simulink model "State_space_validation_lqr_3_5_2_a"  (R2024b)
settings: Solver=FixedStepAuto  StartTime=0.0  StopTime=20  FixedStep=0.001  RelTol=1e-3
undefined symbols (not defined in the file): degs2rpm, DiscIntNeverNeededParam, K, Kff, National_Instruments, PCI, rdp, rpm2rads, sens, step_gain, Ts, u_bar_max
libraries: sldrtlib x3, simulink x1
settings Model: SimulationMode=external  ExtModeTrigDuration=50001  ExtModeTrigDurationFloating=50001  Creator=perondavid  LastModifiedBy=Enrico
settings DataIOCC: LoggingToFile=on
settings OptimizationCC: ReuseModelBlockBuffer=off
settings HardwareCC: ProdBitPerLong=64  ProdHWDeviceType=Intel->x86-64 (Linux 64)
settings RTWCC: Description=Simulink Desktop Real-Time  SystemTargetFile=sldrt.tlc  TemplateMakefile=sldrt.tmf  RTWCompilerOptimization=on  GPUComputeCapability=3.5
settings CodeAppCC: MaxIdLength=95
settings SimulinkDesktopRealTimeCC: TargetLibSuffix=_sldrt.a  TargetPreCompLibLocation=D:\Programmi (D)\MATLAB\R2024b\toolbox\sldrt\lib\win64  ParMdlRefBuildCompliant=on

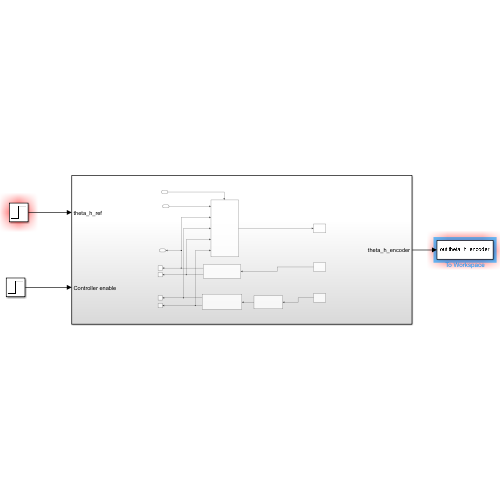
[thumbnail: Simulink's stored preview of the top-level diagram]
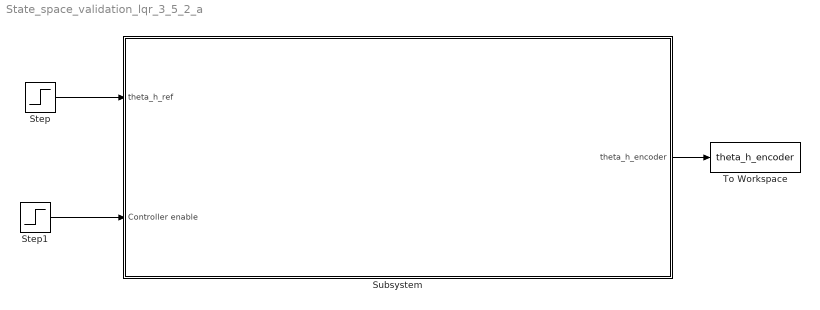
== system State_space_validation_lqr_3_5_2_a ==
  Step : Step  Time=3  After=step_gain  SampleTime=0
  Step1 : Step  Time=2  SampleTime=0
  Subsystem : Subsystem
  To Workspace : ToWorkspace  VariableName=theta_h_encoder  SaveFormat=Structure With Time  SampleTime=Ts
  wires:
  Step/1 -> Subsystem/1(theta_h_ref)
  Step1/1 -> Subsystem/2(Controller enable)
  Subsystem/1(theta_h_encoder) -> To Workspace/1

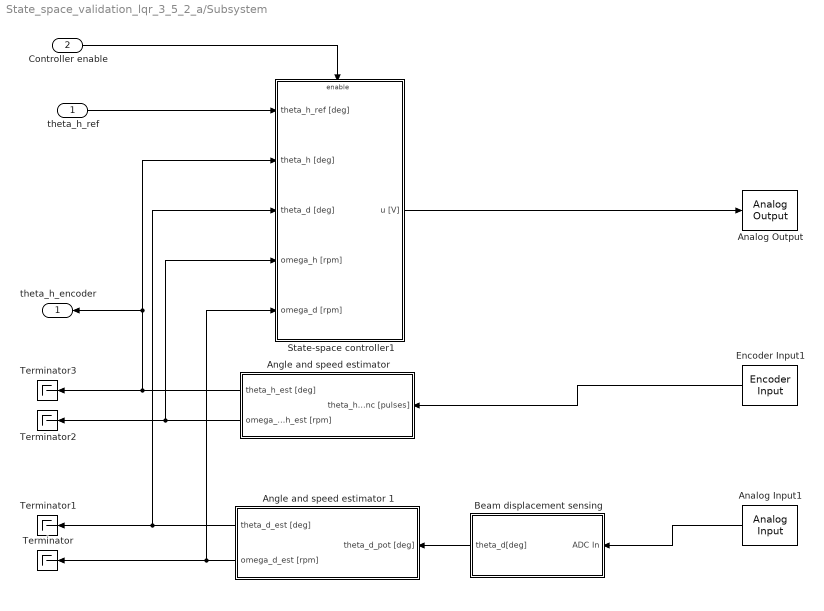
== system State_space_validation_lqr_3_5_2_a/Subsystem ==
  theta_h_ref : Inport
  Controller enable : Inport  Port=2
  Analog Input1 : sldrtlib/Analog Input  SampleTime=-1  MaxMissedTicks=10  ShowMissedTicks=off  YieldWhenWaiting=off  DrvName=National_Instruments/PCI-6221  DrvAddress=4294967295  DrvOptions=[0 0 0 2 0]  Channels=[3, 4]  RangeMode=1  VoltRange=2  DataType=1
      settings: AttributesFormatString=National Instruments\nPCI-6221 [auto]
  Analog Output : sldrtlib/Analog Output  SampleTime=-1  MaxMissedTicks=10  ShowMissedTicks=off  YieldWhenWaiting=off  DrvName=National_Instruments/PCI-6221  DrvAddress=4294967295  DrvOptions=[0 0 0 2 0]  Channels=1  RangeMode=1  VoltRange=1  InitialValue=0  FinalValue=0
      settings: AttributesFormatString=National Instruments\nPCI-6221 [auto]
  Angle and speed estimator : Subsystem
  Angle and speed estimator 1 : Subsystem
  Beam displacement sensing : Subsystem
  Encoder Input1 : sldrtlib/Encoder Input  SampleTime=-1  MaxMissedTicks=10  ShowMissedTicks=off  YieldWhenWaiting=off  DrvName=National_Instruments/PCI-6221  DrvAddress=4294967295  DrvOptions=[0 0 0 2 0]  Channels=1  QuadMode=3  IndexPulse=1  InputFilter=Inf  DataType=1
      settings: AttributesFormatString=National Instruments\nPCI-6221 [auto]
  State-space controller1 : Subsystem
  Terminator{,1..3} (4 alike) : Terminator
  theta_h_encoder : Outport
  wires:
  State-space controller1/1(u [V]) -> Analog Output/1
  Controller enable/1 -> State-space controller1/Enable
  Angle and speed estimator/2(omega_h_est [rpm]) -> State-space controller1/4(omega_h [rpm]), Terminator2/1
  Angle and speed estimator 1/1(theta_d_est [deg]) -> State-space controller1/3(theta_d [deg]), Terminator1/1
  Angle and speed estimator 1/2(omega_d_est [rpm]) -> State-space controller1/5(omega_d [rpm]), Terminator/1
  Beam displacement sensing/1(theta_d[deg]) -> Angle and speed estimator 1/1(theta_d_pot [deg])
  theta_h_ref/1 -> State-space controller1/1(theta_h_ref [deg])
  Angle and speed estimator/1(theta_h_est [deg]) -> State-space controller1/2(theta_h [deg]), theta_h_encoder/1, Terminator3/1
  Encoder Input1/1 -> Angle and speed estimator/1(theta_h_enc [pulses])
  Analog Input1/1 -> Beam displacement sensing/1(ADC In)

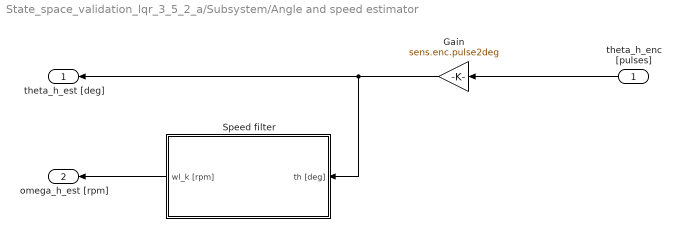
== system State_space_validation_lqr_3_5_2_a/Subsystem/Angle and speed estimator ==
  theta_h_enc [pulses] : Inport
  Gain : Gain  Gain=sens.enc.pulse2deg
  Speed filter : Subsystem
  theta_h_est [deg] : Outport
  omega_h_est [rpm] : Outport  Port=2
  wires:
  Speed filter/1(wl_k [rpm]) -> omega_h_est [rpm]/1
  theta_h_enc [pulses]/1 -> Gain/1
  Gain/1 -> Speed filter/1(th [deg]), theta_h_est [deg]/1

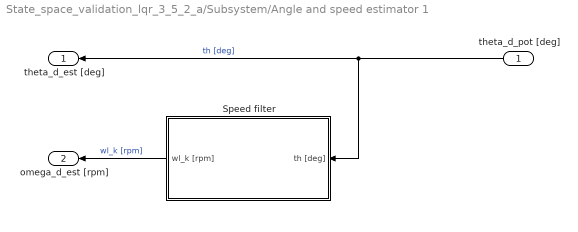
== system State_space_validation_lqr_3_5_2_a/Subsystem/Angle and speed estimator 1 ==
  theta_d_pot [deg] : Inport
  Speed filter : Subsystem
  theta_d_est [deg] : Outport
  omega_d_est [rpm] : Outport  Port=2
  wires:
  Speed filter/1(wl_k [rpm]) -> omega_d_est [rpm]/1  "wl_k [rpm]"
  theta_d_pot [deg]/1 -> Speed filter/1(th [deg]), theta_d_est [deg]/1  "th [deg]"

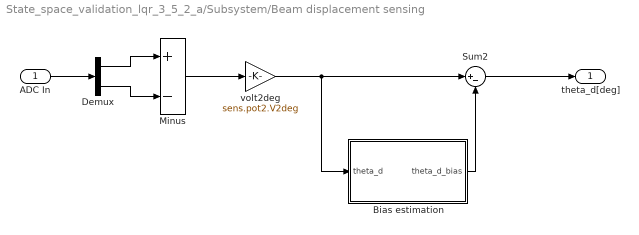
== system State_space_validation_lqr_3_5_2_a/Subsystem/Beam displacement sensing ==
  ADC In : Inport
  " Bias estimation" : Subsystem
  Demux : Demux  Outputs=2
  Minus : Sum  Inputs=+-
  Sum2 : Sum  Inputs=|+-
  volt2deg : Gain  Gain=sens.pot2.V2deg
  theta_d[deg] : Outport
  wires:
  volt2deg/1 -> " Bias estimation"/1(theta_d), Sum2/1
  Sum2/1 -> theta_d[deg]/1
  " Bias estimation"/1(theta_d_bias) -> Sum2/2
  Minus/1 -> volt2deg/1
  Demux/2 -> Minus/2
  ADC In/1 -> Demux/1
  Demux/1 -> Minus/1

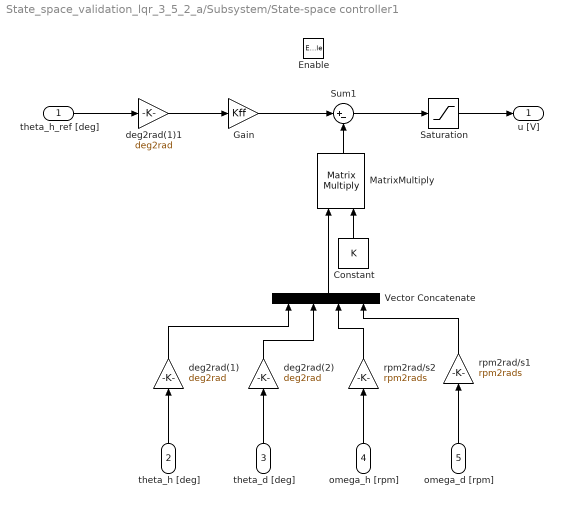
== system State_space_validation_lqr_3_5_2_a/Subsystem/State-space controller1 ==
  theta_h_ref [deg] : Inport
  theta_h [deg] : Inport  Port=2
  theta_d [deg] : Inport  Port=3
  omega_h [rpm] : Inport  Port=4
  omega_d [rpm] : Inport  Port=5
  Enable : EnablePort
  Constant : Constant  Value=K
  Gain : Gain  Gain=Kff
  MatrixMultiply : Product  Multiplication=Matrix(*)
  Saturation : Saturate  UpperLimit=u_bar_max  LowerLimit=-u_bar_max
  Sum1 : Sum  Inputs=|+-
  Vector Concatenate : Concatenate  NumInputs=4
  deg2rad(1) : Gain  Gain=deg2rad
  deg2rad(1)1 : Gain  Gain=deg2rad
  deg2rad(2) : Gain  Gain=deg2rad
  rpm2rad/s1 : Gain  Gain=rpm2rads
  rpm2rad/s2 : Gain  Gain=rpm2rads
  u [V] : Outport
  wires:
  deg2rad(2)/1 -> Vector Concatenate/2
  theta_h [deg]/1 -> deg2rad(1)/1
  Gain/1 -> Sum1/1
  deg2rad(1)/1 -> Vector Concatenate/1
  Constant/1 -> MatrixMultiply/2
  omega_d [rpm]/1 -> rpm2rad/s1/1
  rpm2rad/s2/1 -> Vector Concatenate/3
  rpm2rad/s1/1 -> Vector Concatenate/4
  Vector Concatenate/1 -> MatrixMultiply/1
  MatrixMultiply/1 -> Sum1/2
  theta_d [deg]/1 -> deg2rad(2)/1
  omega_h [rpm]/1 -> rpm2rad/s2/1
  deg2rad(1)1/1 -> Gain/1
  theta_h_ref [deg]/1 -> deg2rad(1)1/1
  Saturation/1 -> u [V]/1
  Sum1/1 -> Saturation/1

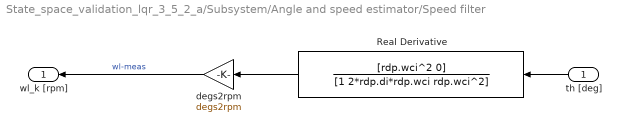
== system State_space_validation_lqr_3_5_2_a/Subsystem/Angle and speed estimator/Speed filter ==
  th [deg] : Inport
  Real Derivative : TransferFcn  Numerator=[rdp.wci^2 0]  Denominator=[1 2*rdp.di*rdp.wci rdp.wci^2]
  degs2rpm : Gain  Gain=degs2rpm
  wl_k [rpm] : Outport
  wires:
  th [deg]/1 -> Real Derivative/1
  degs2rpm/1 -> wl_k [rpm]/1  "wl-meas"
  Real Derivative/1 -> degs2rpm/1

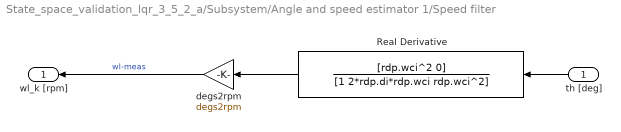
== system State_space_validation_lqr_3_5_2_a/Subsystem/Angle and speed estimator 1/Speed filter ==
  th [deg] : Inport
  Real Derivative : TransferFcn  Numerator=[rdp.wci^2 0]  Denominator=[1 2*rdp.di*rdp.wci rdp.wci^2]
  degs2rpm : Gain  Gain=degs2rpm
  wl_k [rpm] : Outport
  wires:
  th [deg]/1 -> Real Derivative/1
  degs2rpm/1 -> wl_k [rpm]/1  "wl-meas"
  Real Derivative/1 -> degs2rpm/1

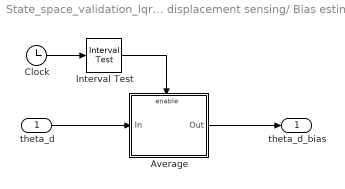
== system State_space_validation_lqr_3_5_2_a/Subsystem/Beam displacement sensing/ Bias estimation ==
  theta_d : Inport
  Average : Subsystem
  Clock : Clock
  Interval Test : simulink/Logic and Bit Operations/Interval Test  IntervalClosedRight=on  uplimit=0.7  IntervalClosedLeft=on  lowlimit=0.2  OutDataTypeStr=boolean
  theta_d_bias : Outport
  wires:
  Clock/1 -> Interval Test/1
  theta_d/1 -> Average/1(In)
  Interval Test/1 -> Average/Enable
  Average/1(Out) -> theta_d_bias/1

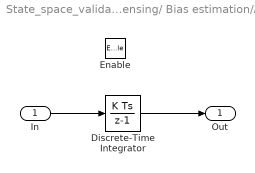
== system State_space_validation_lqr_3_5_2_a/Subsystem/Beam displacement sensing/ Bias estimation/Average ==
  In : Inport
  Enable : EnablePort
  Discrete-Time Integrator : DiscreteIntegrator  SampleTime=Ts  ICPrevOutput=DiscIntNeverNeededParam  ICPrevScaledInput=DiscIntNeverNeededParam
  Out : Outport
  wires:
  In/1 -> Discrete-Time Integrator/1
  Discrete-Time Integrator/1 -> Out/1
